simulink model "MotorImplementation"  (R2022a)
settings: Solver=FixedStepAuto  StartTime=0.0  StopTime=50  FixedStep=1/25  RelTol=1e-3
model workspace (MATLAB code in the model file):
  | %% Mechanical Parameters
  | d_Drum = 23.23e-2; % Meter
  | Drum_Friction = 0.001; % Ns/m
  | Drum_Inertia = 1.0; %kgm^2
  | 
  | n_sh = 5;
  | 
  | %% Load Case 1
  | Hs = 2.2; % m
  | T_w = 8.0; % s
  | m_payload = 8000; % kg
  | h_payload_0 = 75; % m
  | h_payload_final = h_payload_0; % m
  | h_seabed = 350; % m
  | 
  | %% Load Case 2
  | Hs = 2.2; % m
  | T_w = 8.0; % s
  | m_payload = 8000; % kg
  | h_payload_0 = 75; % m
  | h_payload_final = 15; % m
  | h_seabed = 350; % m
  | 
  | %% Load Case 3
  | Hs = 2.2; % m
  | T_w = 8.0; % s
  | m_payload = 8000; % kg
  | h_payload_0 =15; % m
  | h_payload_final = 0; % m
  | h_seabed = 350; % m
  | 
  | %% Sensors
  | % Noise simulation
  | sigma_w = 0.5; %m/s^2 (Standard deviation of noise)
  | beta = 10000; % Positive constant [-]
  | 
  | %% Payload parameters
  | % mass already defined (8000kg)
  | Volume_pl = 2; %m^3
  | Area_pl = 1.5; %m^2
  | C_D = 1.8; %[-] Drag coefficient
  | 
  | %syms rho vel
  | %F_drag = 0.5 * rho * vel^2 * C_D * Area_pl; % Density of sea water(surface) approx 1.025 kg/m^3, velocity comes from the simulation.
  | 
  | %% Seabed
  | k_spring = 1.8e6; %N/m
  | b_damper = 6.5e5; %Ns/m
  | rho = 1.025;
  | %syms delta_x
  | %if delta_x < 0
  | %    F_sb = 0;
  | %else
  | %    F_sb = k_spring*delta_x + b_damper*vel*sqrt(delta_x);
  | %end
  | 
  | %% Bouyant force
  | % The force pushing upwards when something floats down in water. Dependend
  | % on the fluid density, volume of the object falling and gravity
  | g = 9.81;
  | %F_boy = rho * Volume_pl * g;
undefined symbols (not defined in the file or in its folder): I_max, L_M_hat, L_sigma_hat, magnitude, omega_1_N, psi_ref, R_hat, R_R_hat, Ts, V_base, w_BW
libraries: fl_lib x19, nesl_utility x9, CustomComponents_lib x6, simulink x3, slpidlib x2, sdl_lib x1
settings Model: Creator=Jakob  LastModifiedBy=Jakob
settings DebuggingCC: AlgebraicLoopMsg=none

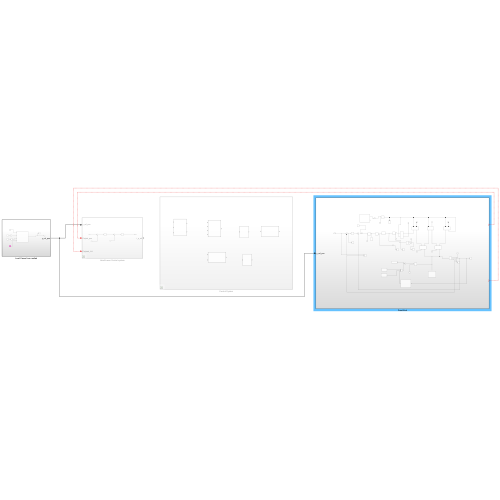
[thumbnail: Simulink's stored preview of the top-level diagram]
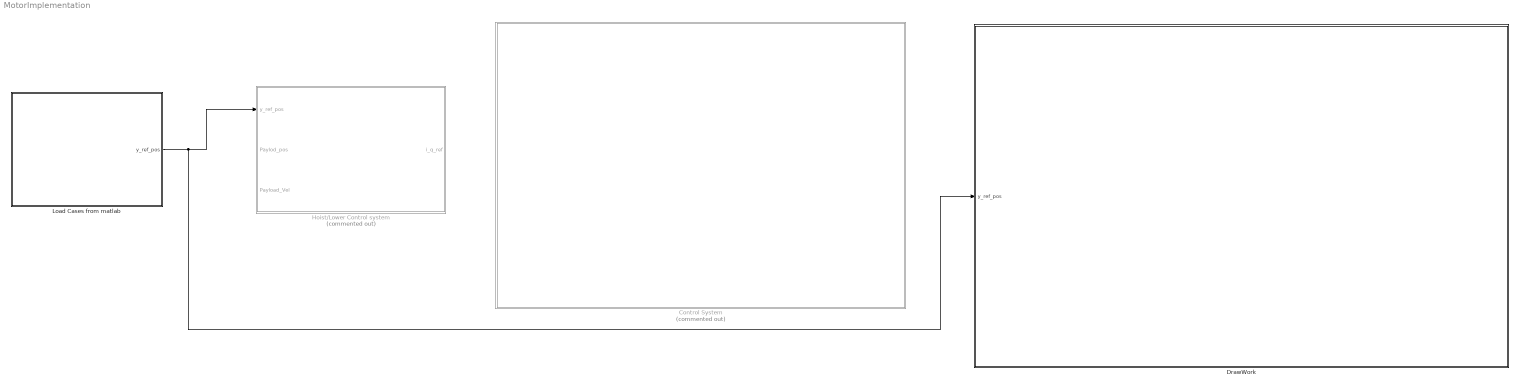
== system MotorImplementation ==
  Control System : Subsystem  Commented=on
  DrawWork : Subsystem
  Hoist/Lower Control system : Subsystem  Commented=on
  Load Cases from matlab : Subsystem
  wires:
  Load Cases from matlab/1(y_ref_pos) -> DrawWork/1(y_ref_pos), Hoist/Lower Control system/1(y_ref_pos)
  ? -> Hoist/Lower Control system/3(Payload_Vel)
  ? -> Hoist/Lower Control system/2(Paylod_pos)

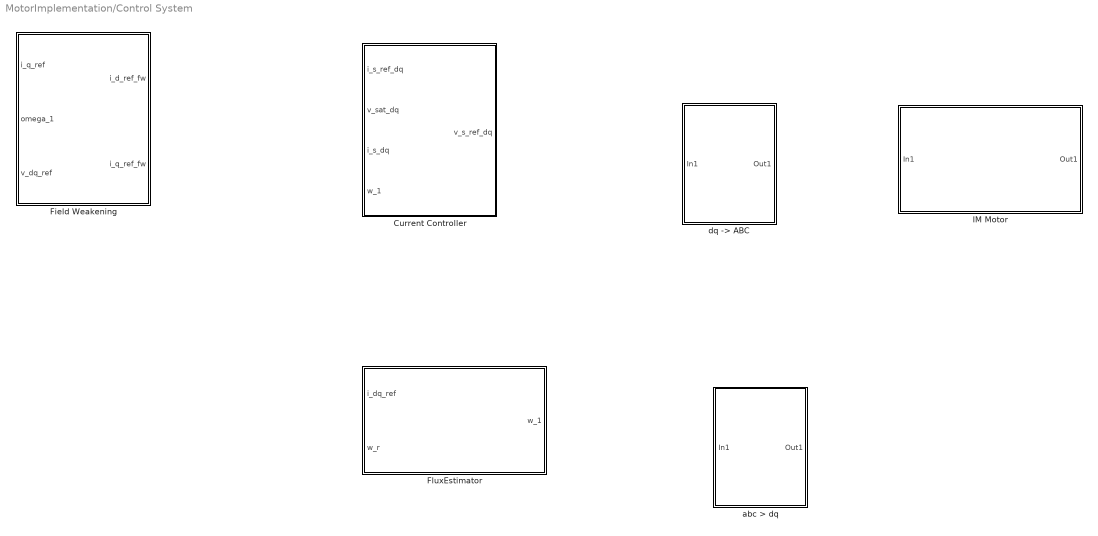
== system MotorImplementation/Control System ==
  Current Controller : Subsystem
  Field Weakening : Subsystem
  FluxEstimator : Subsystem
  IM Motor : Subsystem
  abc > dq : Subsystem
  "dq -> ABC" : Subsystem

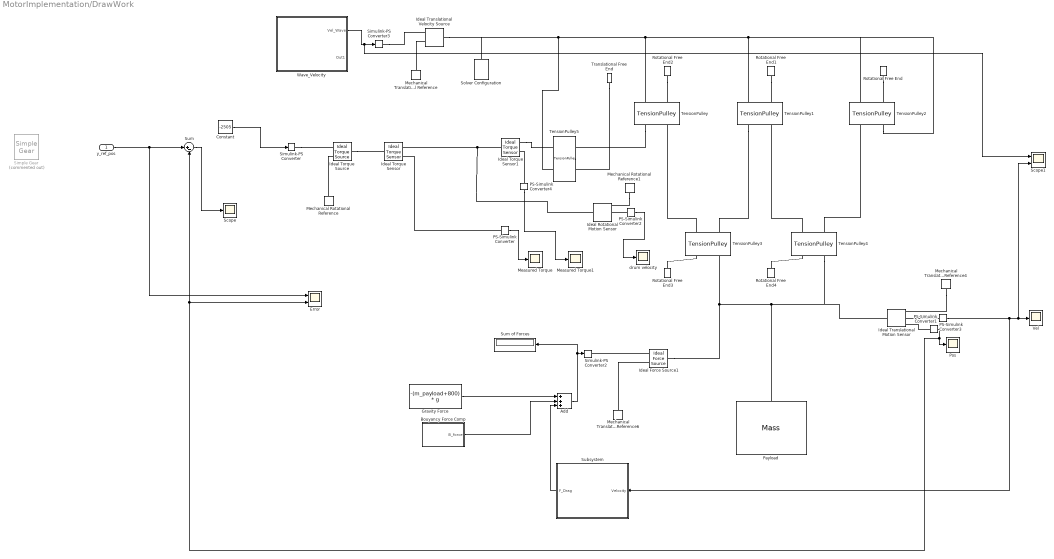
== system MotorImplementation/DrawWork ==
  y_ref_pos : Inport
  Add : Sum  Inputs=+++
  Bouyancy Force Comp : Subsystem
  Constant : Constant  Value=-2505
  Error : Scope  NumInputPorts=2
  Gravity Force : Constant  Value=-(m_payload+800) * g
  Ideal Force Source1 : fl_lib/Mechanical/Mechanical Sources/Ideal Force Source
      settings: SourceProductBaseCode=PW,SS,VE
  Ideal Rotational Motion Sensor : fl_lib/Mechanical/Mechanical Sensors/Ideal Rotational Motion Sensor  wrap_angle=simscape.enum.onoff.off  offset=0 rad
      settings: SourceProductBaseCode=PW,SS,VE
  Ideal Torque Sensor : fl_lib/Mechanical/Mechanical Sensors/Ideal Torque Sensor
      settings: SourceProductBaseCode=PW,SS,VE
  Ideal Torque Sensor1 : fl_lib/Mechanical/Mechanical Sensors/Ideal Torque Sensor
      settings: SourceProductBaseCode=PW,SS,VE
  Ideal Torque Source : fl_lib/Mechanical/Mechanical Sources/Ideal Torque Source
      settings: SourceProductBaseCode=PW,SS,VE
  Ideal Translational Motion Sensor : fl_lib/Mechanical/Mechanical Sensors/Ideal Translational Motion Sensor  offset=70 m
      settings: SourceProductBaseCode=PW,SS,VE
  Ideal Translational Velocity Source : fl_lib/Mechanical/Mechanical Sources/Ideal Translational Velocity Source
      settings: SourceProductBaseCode=PW,SS,VE
  Measured Torque : Scope
  Measured Torque1 : Scope
  Mechanical Rotational Reference : fl_lib/Mechanical/Rotational Elements/Mechanical Rotational Reference
      settings: SourceProductBaseCode=PW,SS,VE
  Mechanical Rotational Reference1 : fl_lib/Mechanical/Rotational Elements/Mechanical Rotational Reference
      settings: SourceProductBaseCode=PW,SS,VE
  Mechanical Translational Reference : fl_lib/Mechanical/Translational Elements/Mechanical Translational Reference
      settings: SourceProductBaseCode=PW,SS,VE
  Mechanical Translational Reference4 : fl_lib/Mechanical/Translational Elements/Mechanical Translational Reference
      settings: SourceProductBaseCode=PW,SS,VE
  Mechanical Translational Reference6 : fl_lib/Mechanical/Translational Elements/Mechanical Translational Reference
      settings: SourceProductBaseCode=PW,SS,VE
  PS-Simulink Converter{,1..4} (5 alike) : nesl_utility/PS-Simulink Converter  PhysicalDomain=network_engine_domain  SubClassName=ps_output  LeftPortType=input  RightPortType=output  PseudoPeriodic=off  Frequencies=[]  VectorFormat=inherit  Unit=inherit  AffineConversion=off
      settings: SourceProductBaseCode=SS,PW,VE
  Payload : fl_lib/Mechanical/Translational Elements/Mass  mass=8800 kg  num_ports=foundation.enum.numPorts2.one  v_specify=off  v_priority=High  v=0 m/s  v_nominal_specify=off  v_nominal_unit=m/s  v_nominal_value=1  f_specify=off  f_priority=None  f=0 N  f_nominal_specify=off  f_nominal_unit=N  f_nominal_value=1
      settings: SourceProductBaseCode=PW,SS,VE
  Pos : Scope
  Rotational Free End{,1..4} (5 alike) : fl_lib/Mechanical/Rotational Elements/Rotational Free End  w_specify=off  w_priority=None  w=0 rad/s  w_nominal_specify=off  w_nominal_unit=rad/s  w_nominal_value=1
      settings: SourceProductBaseCode=PW,SS,VE
  Scope : Scope
  Scope1 : Scope  NumInputPorts=2
  Simple Gear : sdl_lib/Gears/Simple Gear  Commented=on  ratio=1  rotation_direction=sdl.enum.shaftOutputDirection.opposite  friction_model=sdl.enum.gear_efficiencies_load.off  T_noload=0.1 N*m  T_nom=5 N*m  efficiency_nom=0.8  efficiency=0.8  temperature_TLU=[280, 300, 320] K  load_TLU=[1, 5, 10] N*m  efficiency_TLU=[.95, .9, .85]  efficiency_TLU2=[.85, .8, .75; .95, .9, .85; .85, .8, .7]  w_thr=0.01 rad/s  pwr_thr=0.001 W  backlash_model=sdl.enum.backlashModel.Off  backlash_distance=1e-3 mm  x0=0 mm  r_base=0.1 m  hardstop_model=simscape.enum.hardstop.smooth  transition=1e-4 mm  backlash_stiffness=1e7 N/m  backlash_damping=1e6 N*s/m  e=0  v_tol=0.001 m/s  mu_visc=[0, 0] N*m*s/rad  enable_faults=simscape.enum.onoff.off  efficiency_fault=0.05  external_fault=simscape.enum.onoff.off  temporal_fault=simscape.enum.onoff.off  fault_time=5 s  fault_angles=pi / 12 rad  report_fault=simscape.enum.assert.action.none  thermal_mass=50 J/K  temperature_specify=off  temperature_priority=High  temperature=300 K  temperature_nominal_specify=off  temperature_nominal_unit=K  temperature_nominal_value=1  x_backlash_specify=off  x_backlash_priority=None  x_backlash=0 mm  x_backlash_nominal_specify=off  x_backlash_nominal_unit=mm  x_backlash_nominal_value=1  f_hardstop_specify=off  f_hardstop_priority=None  f_hardstop=0 N  f_hardstop_nominal_specify=off  f_hardstop_nominal_unit=N  f_hardstop_nominal_value=1  v_backlash_specify=off  v_backlash_priority=None  v_backlash=0 m/s  v_backlash_nominal_specify=off  v_backlash_nominal_unit=m/s  v_backlash_nominal_value=1
  Simulink-PS Converter : nesl_utility/Simulink-PS Converter  PhysicalDomain=network_engine_domain  SubClassName=ps_input  LeftPortType=input  RightPortType=output  PseudoPeriodic=off  Frequencies=[]  NoiseDistribution=none  NoiseParameters=[]  Unit=1  AffineConversion=off  FilteringAndDerivatives=provide  SimscapeFilterOrder=1  InputFilterTimeConstant=0.001  UdotUserProvided=0
      settings: SourceProductBaseCode=SS,PW,VE
  Simulink-PS Converter2 : nesl_utility/Simulink-PS Converter  PhysicalDomain=network_engine_domain  SubClassName=ps_input  LeftPortType=input  RightPortType=output  PseudoPeriodic=off  Frequencies=[]  NoiseDistribution=none  NoiseParameters=[]  Unit=1  AffineConversion=off  FilteringAndDerivatives=provide  SimscapeFilterOrder=1  InputFilterTimeConstant=0.001  UdotUserProvided=0
      settings: SourceProductBaseCode=SS,PW,VE
  Simulink-PS Converter3 : nesl_utility/Simulink-PS Converter  PhysicalDomain=network_engine_domain  SubClassName=ps_input  LeftPortType=input  RightPortType=output  PseudoPeriodic=off  Frequencies=[]  NoiseDistribution=none  NoiseParameters=[]  Unit=1  AffineConversion=off  FilteringAndDerivatives=filter  SimscapeFilterOrder=2  InputFilterTimeConstant=0.001  UdotUserProvided=0
      settings: SourceProductBaseCode=SS,PW,VE
  Solver Configuration : nesl_utility/Solver Configuration  PhysicalDomain=network_engine_domain  SubClassName=solver  LeftPortType=input  RightPortType=generic  Tones=[]  Harmonics=[]  SimulateNoise=off  Profile=off  UseLocalSampling=off  EnableSwitchedLinearOptims=on  FrequencyDomain=off  UseCCode=off  RelTol=0.001  AbsTol=0.001  MinStep=1e-09  ToWorkspace=off  RevertToSquareIcSolve=off  NumHomotopyIterations=100  PhasorMode=off  PhasorModeNumHarmonics=1  IndexReductionMethod=DerivativeReplacement  DoDC=off  ResidualTolerance=1e-09  UseLocalSolver=off  LocalSolverChoice=NE_BACKWARD_EULER_ADVANCER  LocalSolverSampleTime=0.001  DoFixedCost=off  MaxNonlinIter=3  MaxModeIter=2  ComputeImpulses=off  ImpulseIterations=2  LinearAlgebra=auto  LinearAlgebraNumThread=0  EquationFormulation=NE_TIME_EF  DelaysMemoryBudget=1024  AutomaticFiltering=on  FilteringTimeConstant=0.001  PartitionStorageMethod=AS_NEEDED  PartitionMemoryBudget=1024  PartitionMethod=ROBUST
      settings: SourceProductBaseCode=SS,PW,VE
  Subsystem : Subsystem
  Sum : Sum  Inputs=|+-
  Sum of Forces : Display
  TensionPulley{,1..2,4} (4 alike) : CustomComponents_lib/TensionPulley  radius=0.05 m  b_damp=0 N*m*s/rad  inertia=0.00001 kg*m^2  mass=0.1 kg  mu_s=1  f_A_specify=off  f_A_priority=None  f_A=0 N  f_A_nominal_specify=off  f_A_nominal_unit=N  f_A_nominal_value=1  f_B_specify=off  f_B_priority=None  f_B=0 N  f_B_nominal_specify=off  f_B_nominal_unit=N  f_B_nominal_value=1  f_C_specify=off  f_C_priority=None  f_C=0 N  f_C_nominal_specify=off  f_C_nominal_unit=N  f_C_nominal_value=1  tau_specify=off  tau_priority=None  tau=0 N*m  tau_nominal_specify=off  tau_nominal_unit=N*m  tau_nominal_value=1  w_specify=off  w_priority=None  w=0 rad/s  w_nominal_specify=off  w_nominal_unit=rad/s  w_nominal_value=1  v_specify=off  v_priority=None  v=0 m/s  v_nominal_specify=off  v_nominal_unit=m/s  v_nominal_value=1
      settings: InternalSimscapePortConfiguration="{\"Bottom\":[],\"Left\":[{\"id\":\"C\",\"label\":\"C\",\"type\":\"foundation.mechanical.translational.translational\"},{\"id\":\"S\",\"label\":\"S\",\"type\":\"foundation.mechanical.rotational.rotational\"}],\"Right\":[{\"id\":\"A\",\"label\":\"A\",\"type\":\"foundation.mechanical.translational.translational\"},{\"id\":\"B\",\"label\":\"B\",\"type\":\"foundation.mechanical.translational.translational\"}],\"Top\":[]}"
  TensionPulley3 : CustomComponents_lib/TensionPulley  radius=0.05 m  b_damp=0 N*m*s/rad  inertia=00.00001 kg*m^2  mass=0.1 kg  mu_s=1  f_A_specify=off  f_A_priority=None  f_A=0 N  f_A_nominal_specify=off  f_A_nominal_unit=N  f_A_nominal_value=1  f_B_specify=off  f_B_priority=None  f_B=0 N  f_B_nominal_specify=off  f_B_nominal_unit=N  f_B_nominal_value=1  f_C_specify=off  f_C_priority=None  f_C=0 N  f_C_nominal_specify=off  f_C_nominal_unit=N  f_C_nominal_value=1  tau_specify=off  tau_priority=None  tau=0 N*m  tau_nominal_specify=off  tau_nominal_unit=N*m  tau_nominal_value=1  w_specify=off  w_priority=None  w=0 rad/s  w_nominal_specify=off  w_nominal_unit=rad/s  w_nominal_value=1  v_specify=off  v_priority=None  v=0 m/s  v_nominal_specify=off  v_nominal_unit=m/s  v_nominal_value=1
      settings: InternalSimscapePortConfiguration="{\"Bottom\":[],\"Left\":[{\"id\":\"C\",\"label\":\"C\",\"type\":\"foundation.mechanical.translational.translational\"},{\"id\":\"S\",\"label\":\"S\",\"type\":\"foundation.mechanical.rotational.rotational\"}],\"Right\":[{\"id\":\"A\",\"label\":\"A\",\"type\":\"foundation.mechanical.translational.translational\"},{\"id\":\"B\",\"label\":\"B\",\"type\":\"foundation.mechanical.translational.translational\"}],\"Top\":[]}"
  TensionPulley5 : CustomComponents_lib/TensionPulley  radius=d_Drum/2 m  b_damp=Drum_Friction N*m*s/rad  inertia=Drum_Inertia kg*m^2  mass=0.1 kg  mu_s=1  f_A_specify=off  f_A_priority=None  f_A=0 N  f_A_nominal_specify=off  f_A_nominal_unit=N  f_A_nominal_value=1  f_B_specify=off  f_B_priority=None  f_B=0 N  f_B_nominal_specify=off  f_B_nominal_unit=N  f_B_nominal_value=1  f_C_specify=off  f_C_priority=None  f_C=0 N  f_C_nominal_specify=off  f_C_nominal_unit=N  f_C_nominal_value=1  tau_specify=off  tau_priority=None  tau=0 N*m  tau_nominal_specify=off  tau_nominal_unit=N*m  tau_nominal_value=1  w_specify=off  w_priority=None  w=0 rad/s  w_nominal_specify=off  w_nominal_unit=rad/s  w_nominal_value=1  v_specify=off  v_priority=None  v=0 m/s  v_nominal_specify=off  v_nominal_unit=m/s  v_nominal_value=1
      settings: InternalSimscapePortConfiguration="{\"Bottom\":[],\"Left\":[{\"id\":\"C\",\"label\":\"C\",\"type\":\"foundation.mechanical.translational.translational\"},{\"id\":\"S\",\"label\":\"S\",\"type\":\"foundation.mechanical.rotational.rotational\"}],\"Right\":[{\"id\":\"A\",\"label\":\"A\",\"type\":\"foundation.mechanical.translational.translational\"},{\"id\":\"B\",\"label\":\"B\",\"type\":\"foundation.mechanical.translational.translational\"}],\"Top\":[]}"
  Translational Free End : fl_lib/Mechanical/Translational Elements/Translational Free End  v_specify=off  v_priority=None  v=0 m/s  v_nominal_specify=off  v_nominal_unit=m/s  v_nominal_value=1
      settings: SourceProductBaseCode=PW,SS,VE  InternalSimscapePortConfiguration="{\"Bottom\":[],\"Left\":[{\"id\":\"V\",\"label\":\"\",\"type\":\"foundation.mechanical.translational.translational\"}],\"Right\":[],\"Top\":[]}"
  Vel : Scope
  Wave_Velocity : Subsystem
  drum velocity : Scope
  wires:
  Subsystem/1(F_Drag) -> Add/3
  Bouyancy Force Comp/1(B_force) -> Add/2
  Add/1 -> Sum of Forces/1, Simulink-PS Converter2/1
  PS-Simulink Converter2/1 -> drum velocity/1
  PS-Simulink Converter/1 -> Measured Torque/1
  Wave_Velocity/1(Vel_Wave) -> Scope1/1, Simulink-PS Converter3/1
  PS-Simulink Converter3/1 -> Subsystem/1(Velocity), Scope1/2, Vel/1
  Gravity Force/1 -> Add/1
  PS-Simulink Converter1/1 -> Error/2, Sum/2, Pos/1
  Sum/1 -> Scope/1
  y_ref_pos/1 -> Error/1, Sum/1
  PS-Simulink Converter4/1 -> Measured Torque1/1
  Constant/1 -> Simulink-PS Converter/1
  connections:
  Ideal Torque Source/LConn1 -- Ideal Torque Sensor/LConn1
  TensionPulley4/LConn1 -- Ideal Translational Motion Sensor/LConn1 -- Payload/LConn1 -- TensionPulley3/LConn1 -- Ideal Force Source1/LConn1
  TensionPulley/LConn1 -- TensionPulley2/LConn1 -- TensionPulley2/RConn2 -- TensionPulley1/LConn1 -- TensionPulley5/LConn1 -- Solver Configuration/RConn1 -- Ideal Translational Velocity Source/LConn1
  Rotational Free End3/LConn1 -- TensionPulley3/LConn2
  TensionPulley4/RConn1 -- TensionPulley2/RConn1
  Simulink-PS Converter/RConn1 -- Ideal Torque Source/RConn1
  Ideal Force Source1/RConn1 -- Simulink-PS Converter2/RConn1
  Rotational Free End/LConn1 -- TensionPulley2/LConn2
  Mechanical Rotational Reference1/LConn1 -- Ideal Rotational Motion Sensor/RConn1
  Simulink-PS Converter3/RConn1 -- Ideal Translational Velocity Source/RConn1
  PS-Simulink Converter1/LConn1 -- Ideal Translational Motion Sensor/RConn3
  PS-Simulink Converter2/LConn1 -- Ideal Rotational Motion Sensor/RConn2
  Mechanical Rotational Reference/LConn1 -- Ideal Torque Source/RConn2
  Mechanical Translational Reference6/LConn1 -- Ideal Force Source1/RConn2
  Ideal Rotational Motion Sensor/LConn1 -- Ideal Torque Sensor/RConn1 -- Ideal Torque Sensor1/LConn1
  Rotational Free End4/LConn1 -- TensionPulley4/LConn2
  PS-Simulink Converter3/LConn1 -- Ideal Translational Motion Sensor/RConn2
  TensionPulley3/RConn2 -- TensionPulley/RConn2
  TensionPulley4/RConn2 -- TensionPulley1/RConn2
  Mechanical Translational Reference4/LConn1 -- Ideal Translational Motion Sensor/RConn1
  PS-Simulink Converter/LConn1 -- Ideal Torque Sensor/RConn2
  Rotational Free End1/LConn1 -- TensionPulley1/LConn2
  TensionPulley1/RConn1 -- TensionPulley3/RConn1
  Mechanical Translational Reference/LConn1 -- Ideal Translational Velocity Source/RConn2
  Rotational Free End2/LConn1 -- TensionPulley/LConn2
  TensionPulley/RConn1 -- TensionPulley5/RConn2
  Translational Free End/LConn1 -- TensionPulley5/RConn1
  Ideal Torque Sensor1/RConn1 -- TensionPulley5/LConn2
  PS-Simulink Converter4/LConn1 -- Ideal Torque Sensor1/RConn2

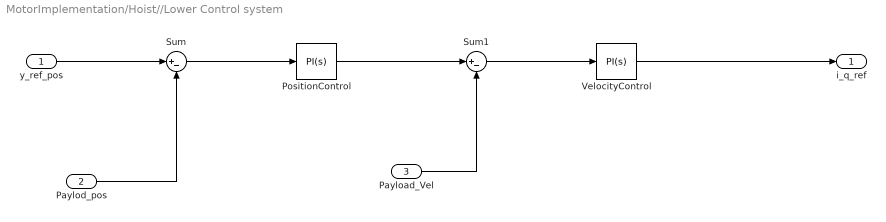
== system MotorImplementation/Hoist//Lower Control system ==
  y_ref_pos : Inport
  Paylod_pos : Inport  Port=2
  Payload_Vel : Inport  Port=3
  PositionControl : slpidlib/PID Controller  Controller=PI  Form=Parallel  TimeDomain=Continuous-time  UseExternalTs=off  SampleTime=-1  IntegratorMethod=Forward Euler  FilterMethod=Forward Euler  ControllerParametersSource=internal  P=1  I=1  UseKiTs=off  D=0  N=100  UseFilter=on  TunerSelectOption=Transfer Function Based (PID Tuner App)  InitialConditionSource=internal  InitialConditionForIntegrator=0  InitialConditionForFilter=0  DifferentiatorICPrevScaledInput=0  ExternalReset=none  TrackingMode=off  Kt=1  LimitOutput=off  SatLimitsSource=internal  UpperSaturationLimit=inf  LowerSaturationLimit=-inf  LinearizeAsGain=on  AntiWindupMode=none  Kb=1  POutMin=[]  POutMax=[]  IOutMin=[]  IOutMax=[]  DOutMin=[]  DOutMax=[]  NOutMin=[]  NOutMax=[]  SumOutMin=[]  SumOutMax=[]  SaturationOutMin=[]  SaturationOutMax=[]  PParamMin=[]  PParamMax=[]  IParamMin=[]  IParamMax=[]  DParamMin=[]  DParamMax=[]  NParamMin=[]  NParamMax=[]  KbParamMin=[]  KbParamMax=[]  KtParamMin=[]  KtParamMax=[]  KbOutMin=[]  KbOutMax=[]  KtOutMin=[]  KtOutMax=[]  IntegratorOutMin=[]  IntegratorOutMax=[]  FilterOutMin=[]  FilterOutMax=[]  SumI1OutMin=[]  SumI1OutMax=[]  SumI2OutMin=[]  SumI2OutMax=[]  SumI3OutMin=[]  SumI3OutMax=[]  SumI4OutMin=[]  SumI4OutMax=[]  SumDOutMin=[]  SumDOutMax=[]  DifferentiatorOutMin=[]  DifferentiatorOutMax=[]  FilterDiffOutCoefMin=[]  FilterDiffOutCoefMax=[]  ReciprocalOutMin=[]  ReciprocalOutMax=[]  SumDenOutMin=[]  SumDenOutMax=[]  SumNumOutMin=[]  SumNumOutMax=[]  DivideOutMin=[]  DivideOutMax=[]  UdiffTsProdOutMin=[]  UdiffTsProdOutMax=[]  NTsProdOutMin=[]  NTsProdOutMax=[]  UintegralTsProdOutMin=[]  UintegralTsProdOutMax=[]  UngainTsProdOutMin=[]  UngainTsProdOutMax=[]  IntegratorContinuousStateAttributes=''  IntegratorStateMustResolveToSignalObject=off  IntegratorRTWStateStorageClass=Auto  FilterContinuousStateAttributes=''  FilterStateMustResolveToSignalObject=off  FilterRTWStateStorageClass=Auto  ParallelPVariant=InternalParameters  IdealPVariant=Disabled  IVariant=InternalParameters  DVariant=Disabled  IntegratorVariant=Continuous  SatVariant=Disabled  AWVariant=Passthrough  PCopyVariant=Disabled  TRVariant=Disabled  FdbkBlocksVariant=Forward  IdealPFdbkVariant=Disabled  SatFdbkVariant=Disabled  DerivativeFilterVariant=Disabled  NVariant=Disabled  NCopyVariant=Disabled_SignalSpec  FilterICVariant=Disabled  IntegratorICVariant=InternalICs  ExternalResetVariant=Disabled  TRSumVariant=Passthrough  SumFdbkVariant=Disabled  SumVariant=Sum_PI  TsampFilterVariant=InternalTs  TsampNgainVariant=Passthrough  TsampIntegralVariant=Passthrough  ExternalSaturationOutDataTypeStr=Inherit: Same as second input  aMode=0
  Sum : Sum  Inputs=|+-
  Sum1 : Sum  Inputs=|+-
  VelocityControl : slpidlib/PID Controller  Controller=PI  Form=Parallel  TimeDomain=Continuous-time  UseExternalTs=off  SampleTime=-1  IntegratorMethod=Forward Euler  FilterMethod=Forward Euler  ControllerParametersSource=internal  P=1  I=1  UseKiTs=off  D=0  N=100  UseFilter=on  TunerSelectOption=Transfer Function Based (PID Tuner App)  InitialConditionSource=internal  InitialConditionForIntegrator=0  InitialConditionForFilter=0  DifferentiatorICPrevScaledInput=0  ExternalReset=none  TrackingMode=off  Kt=1  LimitOutput=off  SatLimitsSource=internal  UpperSaturationLimit=inf  LowerSaturationLimit=-inf  LinearizeAsGain=on  AntiWindupMode=none  Kb=1  POutMin=[]  POutMax=[]  IOutMin=[]  IOutMax=[]  DOutMin=[]  DOutMax=[]  NOutMin=[]  NOutMax=[]  SumOutMin=[]  SumOutMax=[]  SaturationOutMin=[]  SaturationOutMax=[]  PParamMin=[]  PParamMax=[]  IParamMin=[]  IParamMax=[]  DParamMin=[]  DParamMax=[]  NParamMin=[]  NParamMax=[]  KbParamMin=[]  KbParamMax=[]  KtParamMin=[]  KtParamMax=[]  KbOutMin=[]  KbOutMax=[]  KtOutMin=[]  KtOutMax=[]  IntegratorOutMin=[]  IntegratorOutMax=[]  FilterOutMin=[]  FilterOutMax=[]  SumI1OutMin=[]  SumI1OutMax=[]  SumI2OutMin=[]  SumI2OutMax=[]  SumI3OutMin=[]  SumI3OutMax=[]  SumI4OutMin=[]  SumI4OutMax=[]  SumDOutMin=[]  SumDOutMax=[]  DifferentiatorOutMin=[]  DifferentiatorOutMax=[]  FilterDiffOutCoefMin=[]  FilterDiffOutCoefMax=[]  ReciprocalOutMin=[]  ReciprocalOutMax=[]  SumDenOutMin=[]  SumDenOutMax=[]  SumNumOutMin=[]  SumNumOutMax=[]  DivideOutMin=[]  DivideOutMax=[]  UdiffTsProdOutMin=[]  UdiffTsProdOutMax=[]  NTsProdOutMin=[]  NTsProdOutMax=[]  UintegralTsProdOutMin=[]  UintegralTsProdOutMax=[]  UngainTsProdOutMin=[]  UngainTsProdOutMax=[]  IntegratorContinuousStateAttributes=''  IntegratorStateMustResolveToSignalObject=off  IntegratorRTWStateStorageClass=Auto  FilterContinuousStateAttributes=''  FilterStateMustResolveToSignalObject=off  FilterRTWStateStorageClass=Auto  ParallelPVariant=InternalParameters  IdealPVariant=Disabled  IVariant=InternalParameters  DVariant=Disabled  IntegratorVariant=Continuous  SatVariant=Disabled  AWVariant=Passthrough  PCopyVariant=Disabled  TRVariant=Disabled  FdbkBlocksVariant=Forward  IdealPFdbkVariant=Disabled  SatFdbkVariant=Disabled  DerivativeFilterVariant=Disabled  NVariant=Disabled  NCopyVariant=Disabled_SignalSpec  FilterICVariant=Disabled  IntegratorICVariant=InternalICs  ExternalResetVariant=Disabled  TRSumVariant=Passthrough  SumFdbkVariant=Disabled  SumVariant=Sum_PI  TsampFilterVariant=InternalTs  TsampNgainVariant=Passthrough  TsampIntegralVariant=Passthrough  ExternalSaturationOutDataTypeStr=Inherit: Same as second input  aMode=0
  i_q_ref : Outport
  wires:
  y_ref_pos/1 -> Sum/1
  Sum/1 -> PositionControl/1
  PositionControl/1 -> Sum1/1
  Sum1/1 -> VelocityControl/1
  VelocityControl/1 -> i_q_ref/1
  Paylod_pos/1 -> Sum/2
  Payload_Vel/1 -> Sum1/2

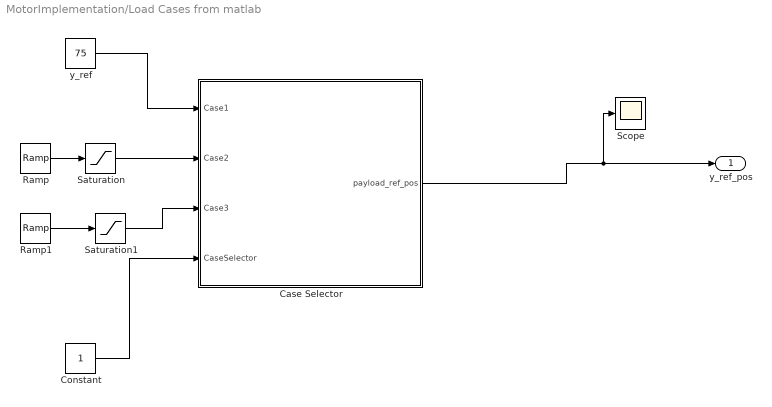
== system MotorImplementation/Load Cases from matlab ==
  Case Selector : MATLAB Function  TreatAsAtomicUnit=on
  Constant : Constant
  Ramp : simulink/Sources/Ramp  slope=-2.5  start=0  InitialOutput=75
  Ramp1 : simulink/Sources/Ramp  slope=-1  start=0  InitialOutput=15
  Saturation : Saturate  UpperLimit=75  LowerLimit=15
  Saturation1 : Saturate  UpperLimit=15  LowerLimit=0
  Scope : Scope
  y_ref : Constant  Value=75
  y_ref_pos : Outport
  wires:
  Case Selector/1(payload_ref_pos) -> Scope/1, y_ref_pos/1
  Constant/1 -> Case Selector/4(CaseSelector)
  y_ref/1 -> Case Selector/1(Case1)
  Ramp/1 -> Saturation/1
  Saturation/1 -> Case Selector/2(Case2)
  Ramp1/1 -> Saturation1/1
  Saturation1/1 -> Case Selector/3(Case3)

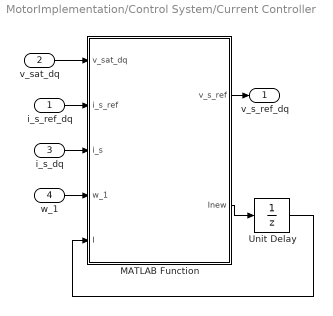
== system MotorImplementation/Control System/Current Controller ==
  i_s_ref_dq : Inport
  v_sat_dq : Inport  Port=2
  i_s_dq : Inport  Port=3
  w_1 : Inport  Port=4
  MATLAB Function : MATLAB Function  TreatAsAtomicUnit=on
  Unit Delay : UnitDelay  SampleTime=-1  HasFrameUpgradeWarning=on
  v_s_ref_dq : Outport  PortDimensions=2
  wires:
  v_sat_dq/1 -> MATLAB Function/1(v_sat_dq)
  Unit Delay/1 -> MATLAB Function/5(I)
  i_s_ref_dq/1 -> MATLAB Function/2(i_s_ref)
  i_s_dq/1 -> MATLAB Function/3(i_s)
  MATLAB Function/2(Inew) -> Unit Delay/1
  w_1/1 -> MATLAB Function/4(w_1)
  MATLAB Function/1(v_s_ref) -> v_s_ref_dq/1

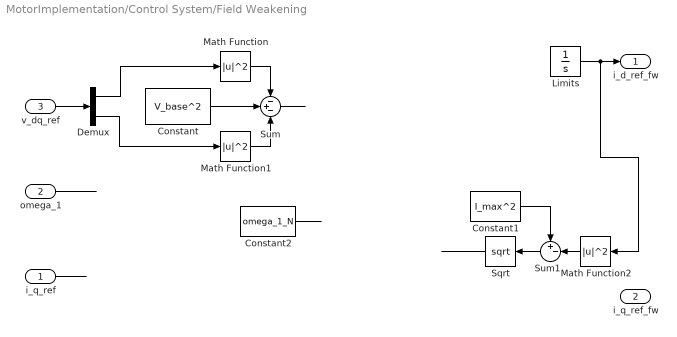
== system MotorImplementation/Control System/Field Weakening ==
  i_q_ref : Inport
  omega_1 : Inport  Port=2
  v_dq_ref : Inport  Port=3
  Constant : Constant  Value=V_base^2
  Constant1 : Constant  Value=I_max^2
  Constant2 : Constant  Value=omega_1_N
  Demux : Demux  Outputs=2
  Limits : Integrator  LimitOutput=on  UpperSaturationLimit=psi_ref/L_M_hat  LowerSaturationLimit=0.1*psi_ref/L_M_hat
  Math Function : Math  Operator=magnitude^2
  Math Function1 : Math  Operator=magnitude^2
  Math Function2 : Math  Operator=magnitude^2
  Sqrt : Sqrt
  Sum : Sum  Inputs=-+-
  Sum1 : Sum  Inputs=+-|
  i_d_ref_fw : Outport
  i_q_ref_fw : Outport  Port=2
  wires:
  Sum/1 -> ?
  ? -> i_q_ref_fw/1
  Constant2/1 -> ?
  ? -> Limits/1
  omega_1/1 -> ?
  Sqrt/1 -> ?
  v_dq_ref/1 -> Demux/1
  i_q_ref/1 -> ?
  Demux/2 -> Math Function1/1
  Constant1/1 -> Sum1/1
  Math Function1/1 -> Sum/3
  Demux/1 -> Math Function/1
  Sum1/1 -> Sqrt/1
  Math Function2/1 -> Sum1/2
  Constant/1 -> Sum/2
  Math Function/1 -> Sum/1
  Limits/1 -> Math Function2/1, i_d_ref_fw/1

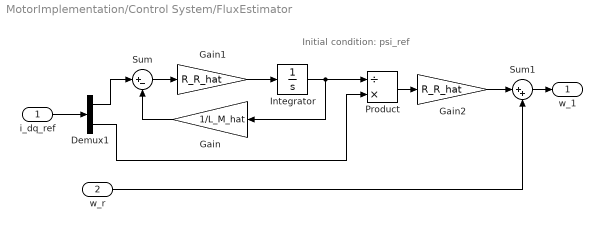
== system MotorImplementation/Control System/FluxEstimator ==
  note: Initial condition: psi_ref
  i_dq_ref : Inport
  w_r : Inport  Port=2
  Demux1 : Demux  Outputs=2
  Gain : Gain  Gain=1/L_M_hat
  Gain1 : Gain  Gain=R_R_hat
  Gain2 : Gain  Gain=R_R_hat
  Integrator : Integrator  InitialCondition=psi_ref
  Product : Product  Inputs=/*
  Sum : Sum  Inputs=|+-
  Sum1 : Sum  Inputs=|++
  w_1 : Outport
  wires:
  Gain/1 -> Sum/2
  Sum/1 -> Gain1/1
  Demux1/1 -> Sum/1
  w_r/1 -> Sum1/2
  Integrator/1 -> Gain/1, Product/1
  Gain2/1 -> Sum1/1
  Product/1 -> Gain2/1
  Gain1/1 -> Integrator/1
  Demux1/2 -> Product/2
  Sum1/1 -> w_1/1
  i_dq_ref/1 -> Demux1/1

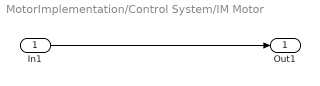
== system MotorImplementation/Control System/IM Motor ==
  In1 : Inport
  Out1 : Outport
  wires:
  In1/1 -> Out1/1

== system MotorImplementation/Control System/abc > dq ==
  In1 : Inport
  Out1 : Outport
  wires:
  In1/1 -> Out1/1

== system MotorImplementation/Control System/dq -> ABC ==
  In1 : Inport
  Out1 : Outport
  wires:
  In1/1 -> Out1/1

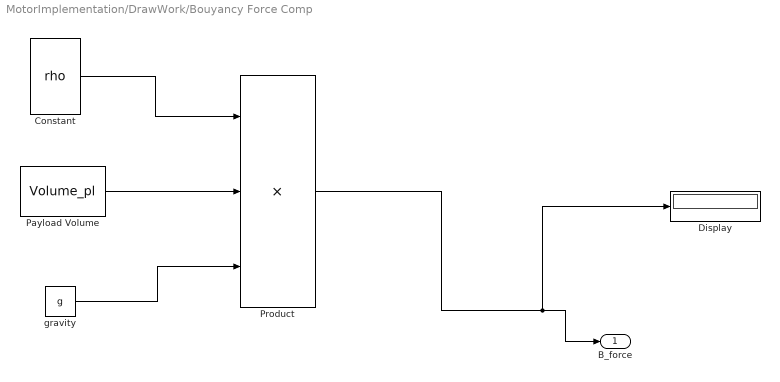
== system MotorImplementation/DrawWork/Bouyancy Force Comp ==
  Constant : Constant  Value=rho
  Display : Display
  Payload Volume : Constant  Value=Volume_pl
  Product : Product  Inputs=3
  gravity : Constant  Value=g
  B_force : Outport
  wires:
  Constant/1 -> Product/1
  Payload Volume/1 -> Product/2
  gravity/1 -> Product/3
  Product/1 -> Display/1, B_force/1

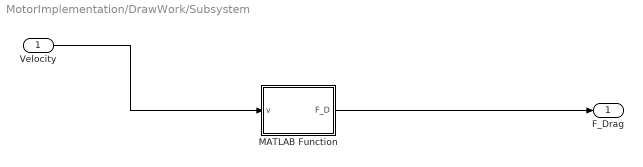
== system MotorImplementation/DrawWork/Subsystem ==
  Velocity : Inport
  MATLAB Function : MATLAB Function  TreatAsAtomicUnit=on
  F_Drag : Outport
  wires:
  Velocity/1 -> MATLAB Function/1(v)
  MATLAB Function/1(F_D) -> F_Drag/1

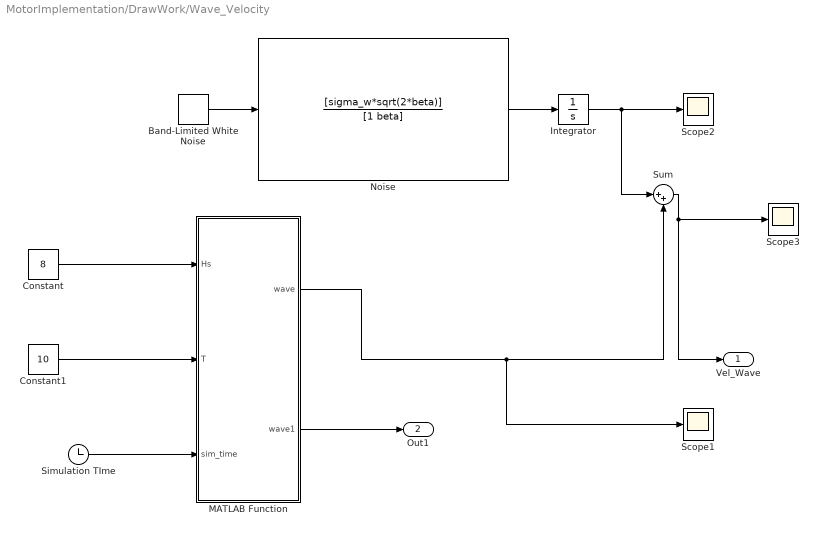
== system MotorImplementation/DrawWork/Wave_Velocity ==
  Band-Limited White Noise : simulink/Sources/Band-Limited White Noise  Cov=[1]  Ts=1/25  seed=[23341]
  Constant : Constant  Value=8
  Constant1 : Constant  Value=10
  Integrator : Integrator
  MATLAB Function : MATLAB Function  TreatAsAtomicUnit=on
  Noise : TransferFcn  Numerator=[sigma_w*sqrt(2*beta)]  Denominator=[1 beta]
  Scope1 : Scope
  Scope2 : Scope
  Scope3 : Scope
  Simulation TIme : Clock
      settings: Decimation=100
  Sum : Sum  Inputs=|++
  Vel_Wave : Outport
  Out1 : Outport  Port=2
  wires:
  Constant/1 -> MATLAB Function/1(Hs)
  Simulation TIme/1 -> MATLAB Function/3(sim_time)
  Constant1/1 -> MATLAB Function/2(T)
  MATLAB Function/1(wave) -> Sum/2, Scope1/1
  Band-Limited White Noise/1 -> Noise/1
  Noise/1 -> Integrator/1
  Sum/1 -> Vel_Wave/1, Scope3/1
  MATLAB Function/2(wave1) -> Out1/1
  Integrator/1 -> Sum/1, Scope2/1

== matlab function MotorImplementation/DrawWork/Wave_Velocity/MATLAB Function ==
  settings: updateMethod=DISCRETE
  data: Hs input; T input; sim_time input; wave output; wave1 output
function [wave, wave1]  = fcn(Hs, T, sim_time)
%WAVE GEN generates stochastic waves
% Hs is the significant wave height [m]
% T is the mean period [s]
% t end is the end time [s]
% t is the time [s]
% wave is sea surface elevation [m]
%% Input parameters
w = linspace (0.1, 2.0, 20); % frequency range
delta_w = w(2) - w(1);
%% PM spectrum (freq. domain )
w1 = (2*pi)/T;
A = 0.11*(Hs^2)*(w1^4);
B = 0.44*(w1^4);
S = (A./w.^5).* exp(-(B./w.^4));
%% Wave amplitude (time domain)
%sfr = 1/25 ; % sampling frequency (Hz) (higher freq −> higher resolution)
t = sim_time; % time vector
phi_test = rng;
phi = 2*pi*(rand(1,length (w))-0.5); % random phase of ith frequency [rad]
rng(phi_test);
A_wave = sqrt(2*S.*delta_w); % amplitude of each sine wave. wave = [] ;

wave1 = [sum(A_wave .*cos(w.*t + phi))];
wave = [sum(A_wave .*-sin(w.*t + phi))];% [m] sea surface elevation  /Derivative

== matlab function MotorImplementation/DrawWork/Subsystem/MATLAB Function ==
  data: v input; F_D output
function F_D = fcn(v)
rho = 1.025;
C_D = 1.8;
Area_pl = 1.5; 


F_D =sign(v) * -(0.5*rho*v^2*C_D*Area_pl);

== matlab function MotorImplementation/Load Cases from matlab/Case Selector ==
  data: Case1 input; Case2 input; Case3 input; CaseSelector input; payload_ref_pos output
function payload_ref_pos  = fcn(Case1, Case2, Case3, CaseSelector)

if CaseSelector == 1
    payload_ref_pos = Case1;
    %select = "Case 1 in progress";
elseif CaseSelector == 2
    payload_ref_pos = Case2;
    %select = "Case 2 in progress";
elseif CaseSelector == 3
    payload_ref_pos = Case3;
    %select = "Case 3 in progress"; 
else 
    payload_ref_pos = 0;
    %select = "No Case is selected";  
end

== matlab function MotorImplementation/Control System/Current Controller/MATLAB Function ==
  data: v_sat_dq input size=2; i_s_ref input size=2; i_s input size=2; w_1 input size=1; I input size=1; w_BW parameter size=1; v_s_ref output size=2; Inew output; R_hat parameter size=1; L_sigma_hat parameter size=1; Ts parameter
function [v_s_ref, Inew] = cc(v_sat_dq,i_s_ref, i_s, w_1, I, w_BW, R_hat, L_sigma_hat, Ts)
%#codegen

%% Current controller 
% Gains
kp = 0; % Complete
ki = 0; % Complete
Ra = 0; % Complete

% Voltage reference in synchronous coordinates
i_s = i_s(1)+ 1i*i_s(2);
i_s_ref = i_s_ref(1)+ 1i*i_s_ref(2);
e = i_s_ref - i_s;
v_s_ref_c = 0; % complete: PI + active resistance Ra + decoupler.
v_s_ref = [real(v_s_ref_c);imag(v_s_ref_c)];

%% Update the integral state of the current controller 
v_sat_dq_c = v_sat_dq(1)+ 1i*v_sat_dq(2);
Inew = I + Ts*(e + (v_sat_dq_c)/kp);
